simulink model "MassSpringKInput"  (R2023b)
settings: Solver=FixedStepAuto  StartTime=0.0  StopTime=60  FixedStep=1  RelTol=1e-3
undefined symbols (not defined in the file): dampingCoefficient, mass
settings Model: ExtModeTrigDuration=100  Creator=20181234  LastModifiedBy=20181234
settings DataIOCC: StateSaveName=tmp_raccel_xout
settings OptimizationCC: EfficientMapNaN2IntZero=off
settings DebuggingCC: ModelReferenceSymbolNameMessage=none
settings HardwareCC: TargetBitPerPointer=64  TargetBitPerSizeT=64  TargetBitPerPtrDiffT=64  TargetLongLongMode=on  TargetIntDivRoundTo=Zero  TargetEndianess=LittleEndian  TargetWordSize=64  TargetHWDeviceType=MATLAB Host  ProdEqTarget=off
settings RTWCC: SystemTargetFile=raccel.tlc  TemplateMakefile=raccel_default_tmf  RTWVerbose=off  RTWUseSimCustomCode=on  CustomBLASCallback=coder.internal.blas.MATLABBLASCallback
settings CodeAppCC: GenerateComments=off  MaxIdLength=128  MangleLength=10  SimulinkBlockComments=off
settings RaccelTargetCC: TargetLangStandard=C99 (ISO)  OptimizeReductions=off  ENABLE_SLEXEC_SSBRIDGE=1  RTWCAPIParams=on  RTWCAPIRootIO=on

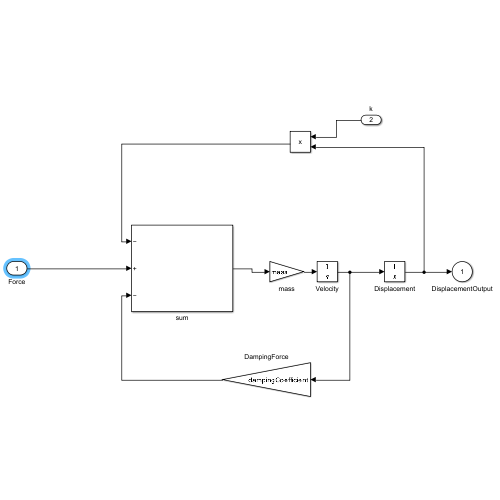
[thumbnail: Simulink's stored preview of the top-level diagram]
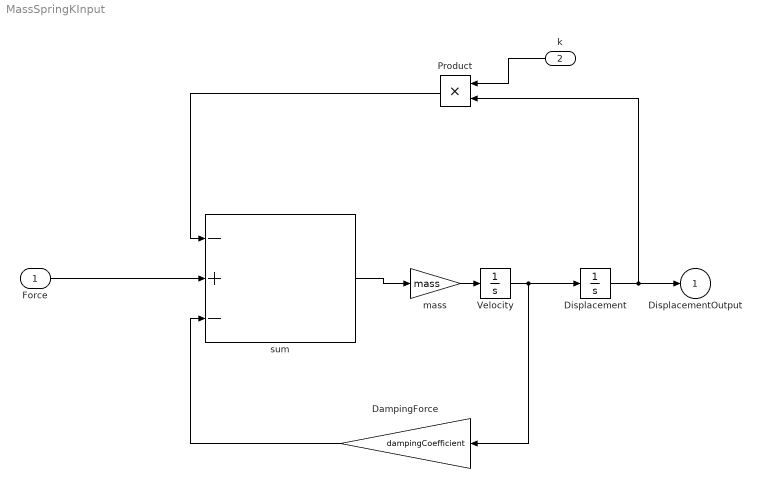
== system MassSpringKInput ==
  Force : Inport
  k : Inport  Port=2
  DampingForce : Gain  Gain=dampingCoefficient
  Displacement : Integrator
  Product : Product
  Velocity : Integrator
  mass : Gain  Gain=mass
  sum : Sum  Inputs=-+-
  DisplacementOutput : Outport
  wires:
  Displacement/1 -> Product/2, DisplacementOutput/1
  Product/1 -> sum/1
  Velocity/1 -> DampingForce/1, Displacement/1
  sum/1 -> mass/1
  DampingForce/1 -> sum/3
  mass/1 -> Velocity/1
  k/1 -> Product/1
  Force/1 -> sum/2
